simulink model "rhszero_aliasing_designed"  (R2014b)
settings: Solver=ode45  StartTime=0.0  StopTime=15  RelTol=1e-3
values from neighbouring files (symbols this model uses):
  aa = exp(-a*h)    [rhszero_variables.m]
  h = 0.05    [BLDC_partial2_fall18.m]    (also in abs_spring18.m = 0.2; active_suspension_ss.m = 0.00416985950901; active_suspension_ss_R.m = 0.00416985950901; active_suspension_ss_spring18.m = 0.004)
  r1 = s0s1r1(3)    [final_dummy.m]
  s0 = 2    [powerplant_dam_controllers.m]
  s1 = -1    [powerplant_dam_controllers.m]
  t0 = subs(Ac, z, 1) / subs(B, z, 1)    [abs_spring18.m]    (also in final_dummy.m = 3.67088607595; harddisk_discrete_design.m = 1/dcgain(Gcb); harddisk_discrete_design_2dof_example.m = 1/dcgain(Gcb))
undefined symbols (not defined in the file or in its folder): r2, r3, s2, s3
libraries: dsparch4 x1, simulink x1
settings Model: Creator=kjartan  LastModifiedBy=kjartan

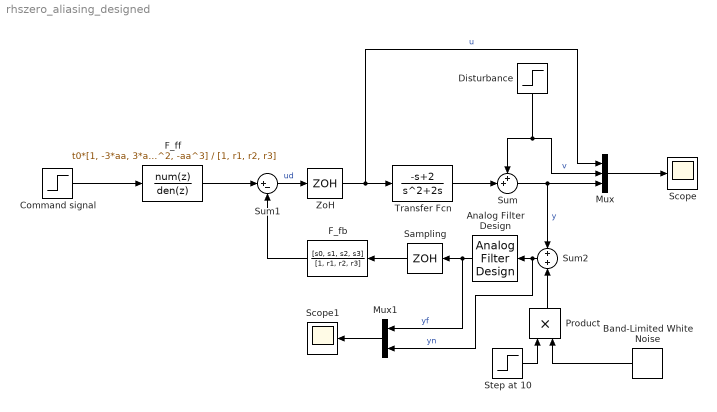
== system rhszero_aliasing_designed ==
  Analog Filter Design : dsparch4/Analog Filter Design  method=Bessel  filttype=Lowpass  N=4  Wlo=1.6*0.3*pi/h  Whi=80  Rp=2  Rs=40
  Band-Limited White Noise : simulink/Sources/Band-Limited White Noise  Cov=[0.01^2]  Ts=0.01  seed=[23341]
  Command signal : Step  Time=0  SampleTime=0
  Disturbance : Step  Time=5  SampleTime=0
  F_fb : DiscreteTransferFcn  Numerator=[s0, s1, s2, s3]  Denominator=[1, r1, r2, r3]  SampleTime=h
  F_ff : DiscreteTransferFcn  Numerator=t0*[1, -3*aa, 3*aa^2, -aa^3]  Denominator=[1, r1, r2, r3]  SampleTime=h
  Mux : Mux  Inputs=3
  Mux1 : Mux  Inputs=2
  Product : Product
  Sampling : ZeroOrderHold  SampleTime=h
  Scope : Scope
      settings: ShowLegends=on
  Scope1 : Scope
      settings: ShowLegends=on
  Step at 10 : Step  Time=10  SampleTime=0
  Sum : Sum  Inputs=++|
  Sum1 : Sum  Inputs=|+-
  Sum2 : Sum  Inputs=+|+
  Transfer Fcn : TransferFcn  Numerator=[-1, 2]  Denominator=[1, 2, 0]
  ZoH : ZeroOrderHold  SampleTime=h
  wires:
  Sum/1 -> Sum2/1, Mux/3  "y"
  Transfer Fcn/1 -> Sum/2
  Mux/1 -> Scope/1
  Command signal/1 -> F_ff/1
  Disturbance/1 -> Sum/1, Mux/2  "v"
  Sum1/1 -> ZoH/1  "ud"
  F_fb/1 -> Sum1/2
  F_ff/1 -> Sum1/1
  ZoH/1 -> Transfer Fcn/1, Mux/1  "u"
  Step at 10/1 -> Product/1
  Band-Limited White Noise/1 -> Product/2
  Product/1 -> Sum2/2
  Sampling/1 -> F_fb/1
  Analog Filter Design/1 -> Mux1/1, Sampling/1  "yf"
  Sum2/1 -> Mux1/2, Analog Filter Design/1  "yn"
  Mux1/1 -> Scope1/1
